simulink model "Simulation_Blocks"  (R2026b)
settings: Solver=VariableStepAuto
libraries: $bdroot x14, fl_lib x7, nesl_utility x6, sm_lib x5, ee_lib x3, simulink x2
settings Model: Creator=Janelyn Anderson  LastModifiedBy=Janelyn Anderson

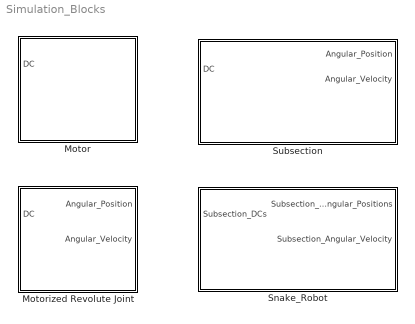
== system Simulation_Blocks ==
  Motor : Subsystem  mask{brake_mode=on}
      mask prompts: brake_mode "Brake Mode Enabled"
  Motorized Revolute Joint : Subsystem  mask{gear_ratio=5}
      mask prompts: gear_ratio "Gear Ratio"
  Snake_Robot : Subsystem
  Subsection : Subsystem

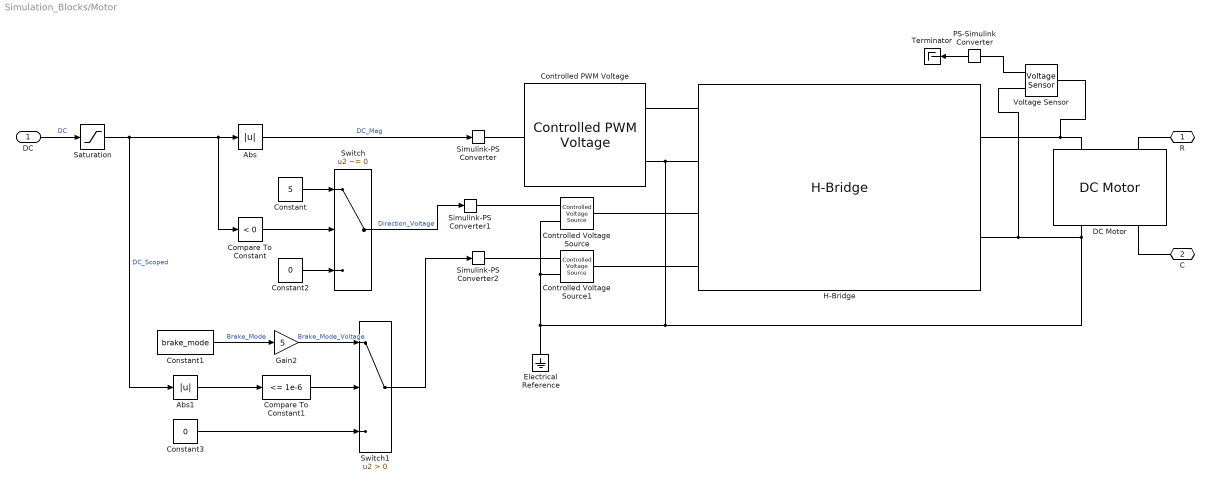
== system Simulation_Blocks/Motor ==
  DC : Inport
  Abs : Abs  SaturateOnIntegerOverflow=off
  Abs1 : Abs  SaturateOnIntegerOverflow=off
  Compare To Constant : simulink/Logic and Bit Operations/Compare To Constant  relop=<  const=0  OutDataTypeStr=boolean
  Compare To Constant1 : simulink/Logic and Bit Operations/Compare To Constant  relop=<=  const=1e-6  OutDataTypeStr=boolean
  Constant : Constant  Value=5
  Constant1 : Constant  Value=brake_mode
  Constant2 : Constant  Value=0
  Constant3 : Constant  Value=0
  Controlled PWM Voltage : ee_lib/Integrated Circuits/Controlled PWM Voltage  F=1000 Hz  TD=0 s  pulse_width_offset=0 s  pulse_min=0 s  pwm_or_av=ee.enum.pwm_or_av.averaged  event_type=ee.enum.ic.event.asynchronous  sample_time=1e-6 s  Vmin=0 V  Vmax=5 V  Vm=5 V  u_min=0  u_max=1
  Controlled Voltage Source : fl_lib/Electrical/Electrical Sources/Controlled Voltage Source
  Controlled Voltage Source1 : fl_lib/Electrical/Electrical Sources/Controlled Voltage Source
  DC Motor : ee_lib/Electromechanical/Brushed Motors/DC Motor  PartSpecification="{\"CollectionId\":\"MW.SimscapeElectrical\",\"CollectionVersion\":\"1.0.0\",\"DatasetId\":\"Faulhaber|3272G_012_CR|simscape.electrical.dcMotor\",\"DisplayName\":\"Faulhaber:3272G_012_CR\"}"  field_option=ee.enum.field_option.pm  Rf=100 % Parameter not set Ohm  Lf=1 % Parameter not set H  Laf=0.15 % Parameter not set H  If0=0 % Parameter not set A  parameterization=ee.enum.dcparam_option.circuit_param  Ra=0.2 % Datasheet derived Ohm  La=0.045 % Datasheet derived mH  emf_or_torque=ee.enum.emf_or_torque.kv  Kv=2.18 % Datasheet derived mV/rpm  Ki=20.81747 % Parameter estimated mN*m/A  T_stall=0.24e-3 % Parameter not set N*m  w_max=19100 % Parameter not set rpm  w_rated=15000 % Parameter not set rpm  P_rated=0.08 % Parameter not set W  V_rated=1.5 % Parameter not set V  lam_param=ee.enum.lam_param.current  i_noload=0.191 % Datasheet derived A  V_i_noload=12 % Datasheet derived V  J=67 % Datasheet derived g*cm^2  lam=0 % % Parameter not set mN*m/(rad/s)  speed0=0 % Parameter not set rpm  alpha=3.93e-3 % Parameter not set 1/K  Tmeas=25 % Parameter not set degC  thermal_mass=138.819875776398 % Parameter estimated J/K  initial_temperature=25 % Parameter not set degC
      settings: AttributesFormatString=Faulhaber:3272G_012_CR
  Electrical Reference : fl_lib/Electrical/Electrical Elements/Electrical Reference
  Gain2 : Gain  Gain=5
  H-Bridge : ee_lib/Semiconductors & Converters/Converters/H-Bridge  supply_ports=ee.enum.supply_ports.hidesupply  pwm_or_av=ee.enum.pwm_or_av.averaged  discontinuous=ee.enum.current_profile.continuous  freewheeling_mode=ee.enum.converters.freewheeling_mode.one_switch_one_diode  Rload=10 Ohm  Lload=1e-5 H  F=10 kHz  regenerative_braking_mode=ee.enum.converters.regenerative_braking_mode.depends_on_rev  Venable=2.5 V  Vmax=5.0 V  Vreverse=2.5 V  Vbrake=2.5 V  Vm=12 V  Ron=0.1 Ohm  Don=0.05 Ohm  Goff=1e-6 S  Tmeas=298.15 K  Ron2=0.1 Ohm  Don2=0.05 Ohm  Tmeas2=398.15 K  thermal_mass=100 J/K  initial_temperature=298.15 K
  PS-Simulink Converter : nesl_utility/PS-Simulink Converter  PhysicalDomain=network_engine_domain  SubClassName=ps_output  LeftPortType=input  RightPortType=output  PseudoPeriodic=off  Frequencies=[]  VectorFormat=inherit  Unit=inherit  AffineConversion=off
  Saturation : Saturate  UpperLimit=1  LowerLimit=-1
  Simulink-PS Converter : nesl_utility/Simulink-PS Converter  PhysicalDomain=network_engine_domain  SubClassName=ps_input  LeftPortType=input  RightPortType=output  PseudoPeriodic=off  Frequencies=[]  NoiseDistribution=none  NoiseParameters=[]  Unit=1  AffineConversion=off  FilteringAndDerivatives=provide  SimscapeFilterOrder=1  InputFilterTimeConstant=0.001  UdotUserProvided=0
  Simulink-PS Converter1 : nesl_utility/Simulink-PS Converter  PhysicalDomain=network_engine_domain  SubClassName=ps_input  LeftPortType=input  RightPortType=output  PseudoPeriodic=off  Frequencies=[]  NoiseDistribution=none  NoiseParameters=[]  Unit=1  AffineConversion=off  FilteringAndDerivatives=provide  SimscapeFilterOrder=1  InputFilterTimeConstant=0.001  UdotUserProvided=0
  Simulink-PS Converter2 : nesl_utility/Simulink-PS Converter  PhysicalDomain=network_engine_domain  SubClassName=ps_input  LeftPortType=input  RightPortType=output  PseudoPeriodic=off  Frequencies=[]  NoiseDistribution=none  NoiseParameters=[]  Unit=1  AffineConversion=off  FilteringAndDerivatives=provide  SimscapeFilterOrder=1  InputFilterTimeConstant=0.001  UdotUserProvided=0
  Switch : Switch  Criteria=u2 ~= 0  SaturateOnIntegerOverflow=off  InputSameDT=off
  Switch1 : Switch  Criteria=u2 > Threshold  SaturateOnIntegerOverflow=off  InputSameDT=off
  Terminator : Terminator
  Voltage Sensor : fl_lib/Electrical/Electrical Sensors/Voltage Sensor
  R : PMIOPort  Side=Right
  C : PMIOPort  Port=2  Side=Left
  wires:
  DC/1 -> Saturation/1  "DC"
  Abs/1 -> Simulink-PS Converter/1  "DC_Mag"
  Saturation/1 -> Abs1/1, Compare To Constant/1, Abs/1  "DC_Scoped"
  Switch/1 -> Simulink-PS Converter1/1  "Direction_Voltage"
  PS-Simulink Converter/1 -> Terminator/1
  Compare To Constant/1 -> Switch/2
  Constant2/1 -> Switch/3
  Constant/1 -> Switch/1
  Constant1/1 -> Gain2/1  "Brake_Mode"
  Gain2/1 -> Switch1/1  "Brake_Mode_Voltage"
  Constant3/1 -> Switch1/3
  Compare To Constant1/1 -> Switch1/2
  Switch1/1 -> Simulink-PS Converter2/1
  Abs1/1 -> Compare To Constant1/1
  connections:
  DC Motor/LConn2 -- R/RConn1
  Controlled Voltage Source1/RConn2 -- Controlled Voltage Source/RConn2 -- Electrical Reference/LConn1 -- Controlled PWM Voltage/RConn2 -- H-Bridge/LConn2 -- DC Motor/RConn1 -- Voltage Sensor/RConn2 -- H-Bridge/RConn2
  Controlled PWM Voltage/RConn1 -- H-Bridge/LConn1
  Simulink-PS Converter2/RConn1 -- Controlled Voltage Source1/RConn1
  Simulink-PS Converter/RConn1 -- Controlled PWM Voltage/LConn1
  H-Bridge/RConn1 -- Voltage Sensor/LConn1 -- DC Motor/LConn1
  Simulink-PS Converter1/RConn1 -- Controlled Voltage Source/RConn1
  DC Motor/RConn2 -- C/RConn1
  Voltage Sensor/RConn1 -- PS-Simulink Converter/LConn1
  H-Bridge/LConn4 -- Controlled Voltage Source1/LConn1
  Controlled Voltage Source/LConn1 -- H-Bridge/LConn3

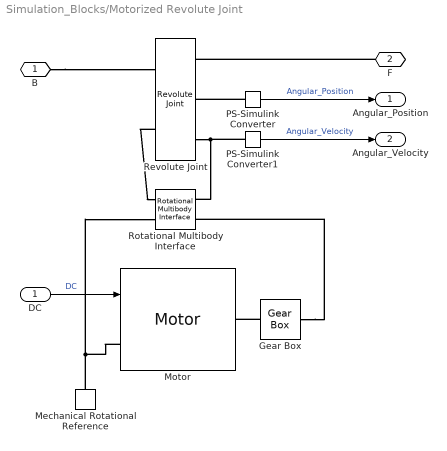
== system Simulation_Blocks/Motorized Revolute Joint ==
  DC : Inport
  Gear Box : fl_lib/Mechanical/Mechanisms/Gear Box  ratio=gear_ratio  t_in_specify=off  t_in_priority=None  t_in=0 N*m  t_in_nominal_specify=off  t_in_nominal_value=1  t_in_nominal_unit=N*m  t_out_specify=off  t_out_priority=None  t_out=0 N*m  t_out_nominal_specify=off  t_out_nominal_value=1  t_out_nominal_unit=N*m
  Mechanical Rotational Reference : fl_lib/Mechanical/Rotational Elements/Mechanical Rotational Reference
  Motor : $bdroot/Motor  brake_mode=on
  PS-Simulink Converter : nesl_utility/PS-Simulink Converter  PhysicalDomain=network_engine_domain  SubClassName=ps_output  LeftPortType=input  RightPortType=output  PseudoPeriodic=off  Frequencies=[]  VectorFormat=inherit  Unit=inherit  AffineConversion=off
  PS-Simulink Converter1 : nesl_utility/PS-Simulink Converter  PhysicalDomain=network_engine_domain  SubClassName=ps_output  LeftPortType=input  RightPortType=output  PseudoPeriodic=off  Frequencies=[]  VectorFormat=inherit  Unit=inherit  AffineConversion=off
  Revolute Joint : sm_lib/Joints/Revolute Joint  JointMode=Normal  CompositeWrenchDir=FollowerOnBase  CompositeWrenchFrame=BaseFrame  SenseConstraintForce=off  SenseConstraintTorque=off  SenseTotalForce=off  SenseTotalTorque=off  PositionTargetSpecify=off  PositionTargetPriority=High  PositionTargetValue=0  PositionTargetValueUnits=deg  VelocityTargetSpecify=off  VelocityTargetPriority=High  VelocityTargetValue=0  VelocityTargetValueUnits=deg/s  EquilibriumPosition=0  EquilibriumPositionUnits=deg  SpringStiffness=0  SpringStiffnessUnits=N*m/deg  DampingCoefficient=0  DampingCoefficientUnits=N*m/(deg/s)  LowerLimitSpecify=on  LowerLimitBound=-90  LowerLimitBoundUnits=deg  LowerLimitStiffness=1e4  LowerLimitStiffnessUnits=N*m/deg  LowerLimitDamping=10  LowerLimitDampingUnits=N*m/(deg/s)  LowerLimitTransitionRegionWidth=0.1  LowerLimitTransitionRegionWidthUnits=deg  UpperLimitSpecify=on  UpperLimitBound=90  UpperLimitBoundUnits=deg  UpperLimitStiffness=1e4  UpperLimitStiffnessUnits=N*m/deg  UpperLimitDamping=10  UpperLimitDampingUnits=N*m/(deg/s)  UpperLimitTransitionRegionWidth=0.1  UpperLimitTransitionRegionWidthUnits=deg  TorqueActuationMode=InputTorque  MotionActuationMode=ComputedMotion  SensePosition=on  SenseVelocity=on  SenseAcceleration=off  SenseTorqueForce=off  SenseLowerLimitTorqueForce=off  SenseUpperLimitTorqueForce=off
  Rotational Multibody Interface : fl_lib/Mechanical/Multibody Interfaces/Rotational Multibody Interface
  B : PMIOPort  Side=Left
  F : PMIOPort  Port=2  Side=Right
  Angular_Position : Outport
  Angular_Velocity : Outport  Port=2
  wires:
  DC/1 -> Motor/1  "DC"
  PS-Simulink Converter/1 -> Angular_Position/1  "Angular_Position"
  PS-Simulink Converter1/1 -> Angular_Velocity/1  "Angular_Velocity"
  connections:
  Motor/LConn1 -- Rotational Multibody Interface/LConn2 -- Mechanical Rotational Reference/LConn1
  Gear Box/LConn1 -- Motor/RConn1
  Gear Box/RConn1 -- Rotational Multibody Interface/RConn2
  Revolute Joint/LConn2 -- Rotational Multibody Interface/LConn1
  Revolute Joint/RConn3 -- Rotational Multibody Interface/RConn1 -- PS-Simulink Converter1/LConn1
  B/RConn1 -- Revolute Joint/LConn1
  F/RConn1 -- Revolute Joint/RConn1
  PS-Simulink Converter/LConn1 -- Revolute Joint/RConn2

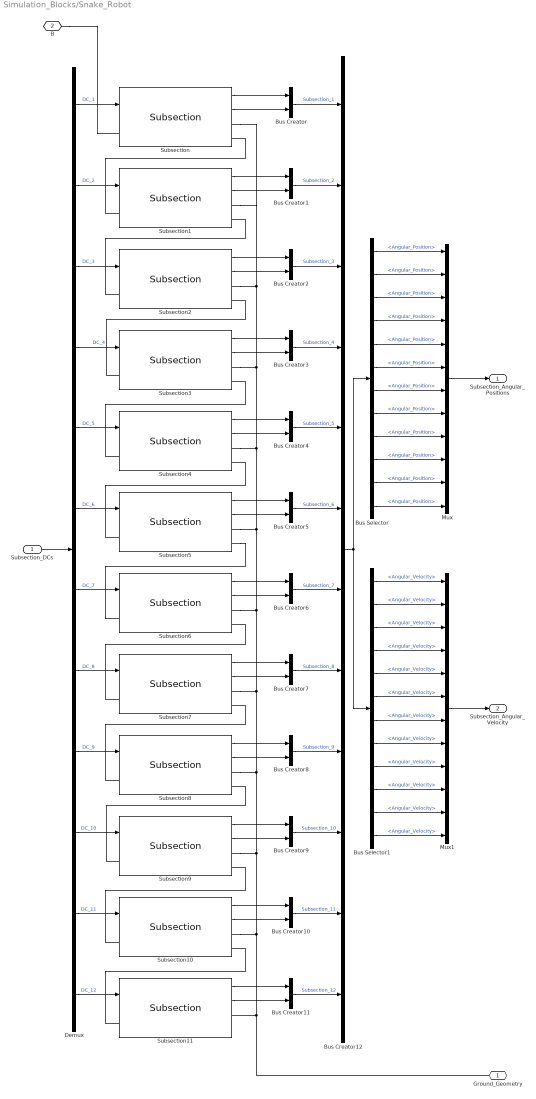
== system Simulation_Blocks/Snake_Robot ==
  Subsection_DCs : Inport
  Bus Creator{,1..11} (12 alike) : BusCreator  Inputs=2
  Bus Creator12 : BusCreator  Inputs=12
  Bus Selector : BusSelector  OutputSignals=Subsection_1.Angular_Position,Subsection_2.Angular_Position,Subsection_3.Angular_Position,Subsection_4.Angular_Position,Subsection_5.Angular_Position,Subsection_6.Angular_Position,Subsection_7.Angular_Position,Subsection_8.Angular_Position,Subsection_9.Angular_Position,Subsection_10.Angular_Position,Subsection_11.Angular_Position,Subsection_12.Angular_Position
  Bus Selector1 : BusSelector  OutputSignals=Subsection_1.Angular_Velocity,Subsection_2.Angular_Velocity,Subsection_3.Angular_Velocity,Subsection_4.Angular_Velocity,Subsection_5.Angular_Velocity,Subsection_6.Angular_Velocity,Subsection_7.Angular_Velocity,Subsection_8.Angular_Velocity,Subsection_9.Angular_Velocity,Subsection_10.Angular_Velocity,Subsection_11.Angular_Velocity,Subsection_12.Angular_Velocity
  Demux : Demux  Outputs=12
  Mux : Mux  Inputs=12
  Mux1 : Mux  Inputs=12
  Subsection{,1..11} (12 alike) : $bdroot/Subsection  SystemSampleTime=-1  VariantActivationTime=update diagram  EmptyChoice=off  PassThrough=off  PassThroughVariantControl=(default)  EmptyChoiceVariantControl=(default)  AllowFlexibleInterface=on  Latency=0  AutoFrameSizeCalculation=off
  Ground_Geometry : PMIOPort  Side=Right
  B : PMIOPort  Port=2  Side=Left
  Subsection_Angular_Positions : Outport
  Subsection_Angular_Velocity : Outport  Port=2
  wires:
  Demux/1 -> Subsection/1  "DC_1"
  Demux/2 -> Subsection1/1  "DC_2"
  Demux/3 -> Subsection2/1  "DC_3"
  Demux/4 -> Subsection3/1  "DC_4"
  Demux/5 -> Subsection4/1  "DC_5"
  Demux/6 -> Subsection5/1  "DC_6"
  Demux/7 -> Subsection6/1  "DC_7"
  Demux/8 -> Subsection7/1  "DC_8"
  Demux/9 -> Subsection8/1  "DC_9"
  Demux/10 -> Subsection9/1  "DC_10"
  Demux/11 -> Subsection10/1  "DC_11"
  Demux/12 -> Subsection11/1  "DC_12"
  Subsection_DCs/1 -> Demux/1
  Subsection/1 -> Bus Creator/1
  Subsection/2 -> Bus Creator/2
  Subsection2/1 -> Bus Creator2/1
  Subsection2/2 -> Bus Creator2/2
  Subsection1/1 -> Bus Creator1/1
  Subsection1/2 -> Bus Creator1/2
  Subsection3/1 -> Bus Creator3/1
  Subsection3/2 -> Bus Creator3/2
  Subsection4/1 -> Bus Creator4/1
  Subsection4/2 -> Bus Creator4/2
  Subsection5/1 -> Bus Creator5/1
  Subsection5/2 -> Bus Creator5/2
  Subsection6/1 -> Bus Creator6/1
  Subsection6/2 -> Bus Creator6/2
  Subsection7/1 -> Bus Creator7/1
  Subsection7/2 -> Bus Creator7/2
  Subsection8/1 -> Bus Creator8/1
  Subsection8/2 -> Bus Creator8/2
  Subsection9/1 -> Bus Creator9/1
  Subsection9/2 -> Bus Creator9/2
  Subsection10/1 -> Bus Creator10/1
  Subsection10/2 -> Bus Creator10/2
  Subsection11/1 -> Bus Creator11/1
  Subsection11/2 -> Bus Creator11/2
  Bus Creator/1 -> Bus Creator12/1  "Subsection_1"
  Bus Creator1/1 -> Bus Creator12/2  "Subsection_2"
  Bus Creator2/1 -> Bus Creator12/3  "Subsection_3"
  Bus Creator3/1 -> Bus Creator12/4  "Subsection_4"
  Bus Creator4/1 -> Bus Creator12/5  "Subsection_5"
  Bus Creator5/1 -> Bus Creator12/6  "Subsection_6"
  Bus Creator6/1 -> Bus Creator12/7  "Subsection_7"
  Bus Creator7/1 -> Bus Creator12/8  "Subsection_8"
  Bus Creator8/1 -> Bus Creator12/9  "Subsection_9"
  Bus Creator9/1 -> Bus Creator12/10  "Subsection_10"
  Bus Creator10/1 -> Bus Creator12/11  "Subsection_11"
  Bus Creator11/1 -> Bus Creator12/12  "Subsection_12"
  Bus Creator12/1 -> Bus Selector/1, Bus Selector1/1
  Bus Selector/1 -> Mux/1  "<Angular_Position>"
  Bus Selector/2 -> Mux/2  "<Angular_Position>"
  Bus Selector/3 -> Mux/3  "<Angular_Position>"
  Bus Selector/4 -> Mux/4  "<Angular_Position>"
  Bus Selector/5 -> Mux/5  "<Angular_Position>"
  Bus Selector/6 -> Mux/6  "<Angular_Position>"
  Bus Selector/7 -> Mux/7  "<Angular_Position>"
  Bus Selector/8 -> Mux/8  "<Angular_Position>"
  Bus Selector/9 -> Mux/9  "<Angular_Position>"
  Bus Selector/10 -> Mux/10  "<Angular_Position>"
  Bus Selector/11 -> Mux/11  "<Angular_Position>"
  Bus Selector/12 -> Mux/12  "<Angular_Position>"
  Mux/1 -> Subsection_Angular_Positions/1
  Mux1/1 -> Subsection_Angular_Velocity/1
  Bus Selector1/1 -> Mux1/1  "<Angular_Velocity>"
  Bus Selector1/2 -> Mux1/2  "<Angular_Velocity>"
  Bus Selector1/3 -> Mux1/3  "<Angular_Velocity>"
  Bus Selector1/4 -> Mux1/4  "<Angular_Velocity>"
  Bus Selector1/5 -> Mux1/5  "<Angular_Velocity>"
  Bus Selector1/6 -> Mux1/6  "<Angular_Velocity>"
  Bus Selector1/7 -> Mux1/7  "<Angular_Velocity>"
  Bus Selector1/8 -> Mux1/8  "<Angular_Velocity>"
  Bus Selector1/9 -> Mux1/9  "<Angular_Velocity>"
  Bus Selector1/10 -> Mux1/10  "<Angular_Velocity>"
  Bus Selector1/11 -> Mux1/11  "<Angular_Velocity>"
  Bus Selector1/12 -> Mux1/12  "<Angular_Velocity>"
  connections:
  Subsection1/LConn1 -- Subsection/RConn2
  Subsection2/LConn1 -- Subsection1/RConn2
  Subsection3/LConn1 -- Subsection2/RConn2
  Subsection4/LConn1 -- Subsection3/RConn2
  Subsection5/LConn1 -- Subsection4/RConn2
  Subsection10/LConn1 -- Subsection9/RConn2
  Subsection7/LConn1 -- Subsection6/RConn2
  Subsection9/LConn1 -- Subsection8/RConn2
  Subsection8/LConn1 -- Subsection7/RConn2
  Subsection11/LConn1 -- Subsection10/RConn2
  Subsection5/RConn2 -- Subsection6/LConn1
  Ground_Geometry/RConn1 -- Subsection/RConn1 -- Subsection1/RConn1 -- Subsection2/RConn1 -- Subsection3/RConn1 -- Subsection4/RConn1 -- Subsection5/RConn1 -- Subsection6/RConn1 -- Subsection7/RConn1 -- Subsection8/RConn1 -- Subsection9/RConn1 -- Subsection10/RConn1 -- Subsection11/RConn1
  B/RConn1 -- Subsection/LConn1

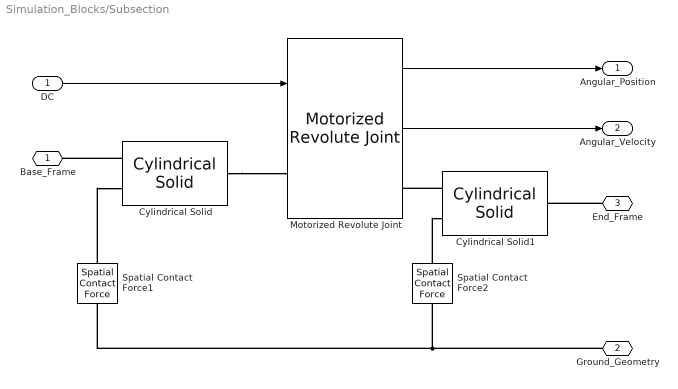
== system Simulation_Blocks/Subsection ==
  DC : Inport
  Cylindrical Solid : sm_lib/Body Elements/Cylindrical Solid  CylinderRadius=2  CylinderRadiusUnits=in  CylinderLength=1.5  CylinderLengthUnits=in  ExportEntireGeometry=on  InertiaType=Custom  BasedOnType=Density  Density=1000  DensityUnits=kg/m^3  Mass=0.5  MassUnits=lbm  CenterOfMass=[0 0 0]  CenterOfMassUnits=m  MomentsOfInertia=[1 1 1]  MomentsOfInertiaUnits=kg*m^2  ProductsOfInertia=[0 0 0]  ProductsOfInertiaUnits=kg*m^2  GraphicType=FromGeometry  MarkerShape=Sphere  MarkerSize=10  GraphicVisPropType=SimpleVisualProperties  GraphicDiffuseColor=[0.8157 0.2471 0.8353]  GraphicOpacity=1  GraphicSpecularColor=[0.5 0.5 0.5 1.0]  GraphicAmbientColor=[0.15 0.15 0.15 1.0]  GraphicEmissiveColor=[0.0 0.0 0.0 1.0]  GraphicShininess=75  DoExposeReferenceFrame=off  SerializedFrames=<Frames><Frame><Id>Frame1</Id><Value><Name>Base Frame</Name><Origin><Source>GeometricFeature</Source><FeatureName>bottom surface</FeatureName></Origin><PrimaryAxis><DefinedDirection>+Z</DefinedDirection><Source>ReferenceFrame</Source><SourceDirection>+Z</SourceDirection><FeatureName></FeatureName></PrimaryAxis><SecondaryAxis><DefinedDirection>+X</DefinedDirection><Source>ReferenceFrame</Source><SourceDirection>+Y</SourceDirection><FeatureName></FeatureName></SecondaryAxis></Value></Frame><Frame><Id>Frame2</Id><Value><Name>End Frame</Name><Origin><Source>GeometricFeature</Source><FeatureName>top surface</FeatureName></Origin><PrimaryAxis><DefinedDirection>+Z</DefinedDirection><Source>ReferenceFrame</Source><SourceDirection>-X</SourceDirection><FeatureName></FeatureName></PrimaryAxis><SecondaryAxis><DefinedDirection>+Y</DefinedDirection><Source>ReferenceFrame</Source><SourceDirection>+Y</SourceDirection><FeatureName></FeatureName></SecondaryAxis></Value></Frame></Frames>
  Cylindrical Solid1 : sm_lib/Body Elements/Cylindrical Solid  CylinderRadius=2  CylinderRadiusUnits=in  CylinderLength=0.5  CylinderLengthUnits=in  ExportEntireGeometry=on  InertiaType=Custom  BasedOnType=Density  Density=1000  DensityUnits=kg/m^3  Mass=0.1  MassUnits=lbm  CenterOfMass=[0 0 0]  CenterOfMassUnits=m  MomentsOfInertia=[1 1 1]  MomentsOfInertiaUnits=kg*m^2  ProductsOfInertia=[0 0 0]  ProductsOfInertiaUnits=kg*m^2  GraphicType=FromGeometry  MarkerShape=Sphere  MarkerSize=10  GraphicVisPropType=SimpleVisualProperties  GraphicDiffuseColor=[0.2431 0.3216 0.8353]  GraphicOpacity=1  GraphicSpecularColor=[0.5 0.5 0.5 1.0]  GraphicAmbientColor=[0.15 0.15 0.15 1.0]  GraphicEmissiveColor=[0.0 0.0 0.0 1.0]  GraphicShininess=75  DoExposeReferenceFrame=off  SerializedFrames=<Frames><Frame><Id>Frame1</Id><Value><Name>Base Frame</Name><Origin><Source>GeometricFeature</Source><FeatureName>bottom surface</FeatureName></Origin><PrimaryAxis><DefinedDirection>+Z</DefinedDirection><Source>ReferenceFrame</Source><SourceDirection>-X</SourceDirection><FeatureName></FeatureName></PrimaryAxis><SecondaryAxis><DefinedDirection>+Y</DefinedDirection><Source>ReferenceFrame</Source><SourceDirection>+Y</SourceDirection><FeatureName></FeatureName></SecondaryAxis></Value></Frame><Frame><Id>Frame2</Id><Value><Name>End Frame</Name><Origin><Source>GeometricFeature</Source><FeatureName>top surface</FeatureName></Origin><PrimaryAxis><DefinedDirection>+Z</DefinedDirection><Source>ReferenceFrame</Source><SourceDirection>+Z</SourceDirection><FeatureName></FeatureName></PrimaryAxis><SecondaryAxis><DefinedDirection>+X</DefinedDirection><Source>ReferenceFrame</Source><SourceDirection>+X</SourceDirection><FeatureName></FeatureName></SecondaryAxis></Value></Frame></Frames>
  Motorized Revolute Joint : $bdroot/Motorized Revolute Joint  gear_ratio=5
  Spatial Contact Force1 : sm_lib/Forces and Torques/Spatial Contact Force  SenseSeparationDistance=off  NormalForceType=SmoothSpringDamper  NormalStiffness=1e6  NormalStiffnessUnits=N/m  NormalDamping=1e3  NormalDampingUnits=N/(m/s)  NormalTransitionRegionWidth=1e-4  NormalTransitionRegionWidthUnits=m  FrictionType=SmoothStickSlip  CoefficientOfStaticFriction=0.5  CoefficientOfDynamicFriction=0.3  FrictionalCriticalVelocity=1e-3  FrictionalCriticalVelocityUnits=m/s  SenseContactSignal=off  SensePenetrationDepth=off  SenseNormalVelocity=off  SenseTangentialVelocity=off  SensingForceTorqueDirection=BaseOnFollower  SensingForceTorqueResolutionFrame=ContactFrame  SenseNormalForce=off  SenseNormalForceMagnitude=off  SenseNormalTorque=off  SenseFrictionalForce=off  SenseFrictionalForceMagnitude=off  SenseFrictionalTorque=off  SenseTotalForce=off  SenseTotalTorque=off  SenseContactBaseRotation=off  SenseContactBaseTranslation=off  SenseContactFollowerRotation=off  SenseContactFollowerTranslation=off  ZeroCrossDetectContactStartAndEnd=off
  Spatial Contact Force2 : sm_lib/Forces and Torques/Spatial Contact Force  SenseSeparationDistance=off  NormalForceType=SmoothSpringDamper  NormalStiffness=1e6  NormalStiffnessUnits=N/m  NormalDamping=1e3  NormalDampingUnits=N/(m/s)  NormalTransitionRegionWidth=1e-4  NormalTransitionRegionWidthUnits=m  FrictionType=SmoothStickSlip  CoefficientOfStaticFriction=0.5  CoefficientOfDynamicFriction=0.3  FrictionalCriticalVelocity=1e-3  FrictionalCriticalVelocityUnits=m/s  SenseContactSignal=off  SensePenetrationDepth=off  SenseNormalVelocity=off  SenseTangentialVelocity=off  SensingForceTorqueDirection=BaseOnFollower  SensingForceTorqueResolutionFrame=ContactFrame  SenseNormalForce=off  SenseNormalForceMagnitude=off  SenseNormalTorque=off  SenseFrictionalForce=off  SenseFrictionalForceMagnitude=off  SenseFrictionalTorque=off  SenseTotalForce=off  SenseTotalTorque=off  SenseContactBaseRotation=off  SenseContactBaseTranslation=off  SenseContactFollowerRotation=off  SenseContactFollowerTranslation=off  ZeroCrossDetectContactStartAndEnd=off
  Base_Frame : PMIOPort  Side=Left
  Ground_Geometry : PMIOPort  Port=2  Side=Right
  End_Frame : PMIOPort  Port=3  Side=Right
  Angular_Position : Outport
  Angular_Velocity : Outport  Port=2
  wires:
  DC/1 -> Motorized Revolute Joint/1
  Motorized Revolute Joint/2 -> Angular_Velocity/1
  Motorized Revolute Joint/1 -> Angular_Position/1
  connections:
  Cylindrical Solid/LConn1 -- Base_Frame/RConn1
  Cylindrical Solid/RConn1 -- Motorized Revolute Joint/LConn1
  Cylindrical Solid1/LConn1 -- Motorized Revolute Joint/RConn1
  Spatial Contact Force1/LConn1 -- Cylindrical Solid/LConn2
  Spatial Contact Force2/LConn1 -- Cylindrical Solid1/LConn2
  End_Frame/RConn1 -- Cylindrical Solid1/RConn1
  Ground_Geometry/RConn1 -- Spatial Contact Force1/RConn1 -- Spatial Contact Force2/RConn1
